simulink model "mecha_discrete_testing"  (R2016b)
settings: Solver=ode1  StartTime=0.0  StopTime=50  FixedStep=0.01  RelTol=1e-3
undefined symbols (not defined in the file or in its folder): DiscIntNeverNeededParam
libraries: dspinverses x1
settings Model: Creator=Utente  LastModifiedBy=Utente

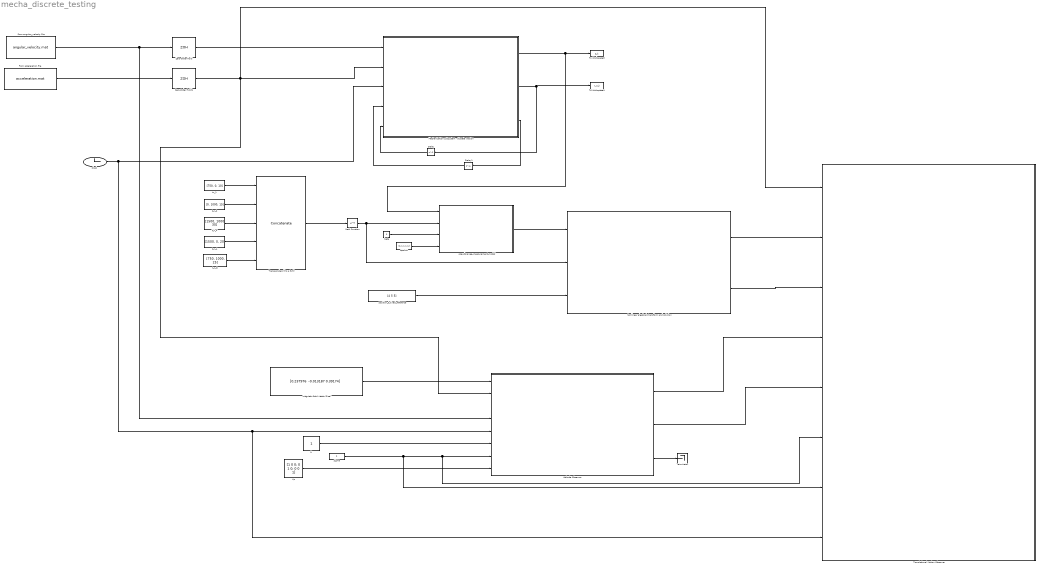
== system mecha_discrete_testing ==
  Attitude Observer : Subsystem
  Clock : Clock
      settings: Decimation=50
  Delay : Delay  DelayLength=1
  Delay1 : Delay  DelayLength=1
  From acceleration file : FromFile  FileName=acceleration.mat  SampleTime=0
  From angular_velocity file : FromFile  FileName=angular_velocity.mat  SampleTime=0
  Kp : Constant  Value=[1 0 0; 0 1 0; 0 0 1]
  Math Function : Math  Operator=transpose  SaturateOnIntegerOverflow=on
  Mechanisation subsystem - discrete version : Subsystem
  Nonlinear algebraic transform and solution : Subsystem
  Terminator : Terminator
  To Workspace3 : ToWorkspace  VariableName=p_k  SaveFormat=Timeseries  SampleTime=-1
  To Workspace4 : ToWorkspace  VariableName=v_n_k  SaveFormat=Timeseries  SampleTime=-1
  Translational Motion Observer : Subsystem
  Transponders (it's a 3x5) : Concatenate  NumInputs=5  Mode=Multidimensional array  ConcatenateDimension=2
  Zero-Order Hold : ZeroOrderHold  SampleTime=0.01
  Zero-Order Hold1 : ZeroOrderHold  SampleTime=0.01
  beta : Constant
  epsilon : Constant  Value=[1 1 1 1 1]
  ki : Constant
  magnetic field vector (Pisa) : Constant  Value="[0.237976  -0.013187 0.39174]"
  position_0_fixed_reference : Constant  Value=[4 5 5]
  pseudorange_measurement_model : MATLAB Function  TreatAsAtomicUnit=on
  sigma : Constant
  t_n_2 : Constant  Value=[0, 1000, 15]
  t_n_3 : Constant  Value=[1500, 1000, 30]
  t_n_4 : Constant  Value=[1500, 0, 20]
  t_n_5 : Constant  Value=[750, 1000, 25]
  tn_1 : Constant  Value=[750, 0, 10]
  wires:
  From acceleration file/1 -> Zero-Order Hold1/1
  From angular_velocity file/1 -> Attitude Observer/4(w_ib), Zero-Order Hold/1
  Zero-Order Hold/1 -> Mechanisation subsystem - discrete version/1(w_ib)
  Mechanisation subsystem - discrete version/1(p_n_k) -> pseudorange_measurement_model/1(p_n), To Workspace3/1
  Mechanisation subsystem - discrete version/3(R_nb_k_1) -> Delay1/1
  Mechanisation subsystem - discrete version/2(v_n_k_1) -> Delay/1, To Workspace4/1
  Delay/1 -> Mechanisation subsystem - discrete version/5(v_n_k)
  Delay1/1 -> Mechanisation subsystem - discrete version/4(R_nb_k)
  beta/1 -> pseudorange_measurement_model/3(beta)
  epsilon/1 -> pseudorange_measurement_model/4(epsilon)
  t_n_5/1 -> Transponders (it's a 3x5)/5
  t_n_4/1 -> Transponders (it's a 3x5)/4
  t_n_3/1 -> Transponders (it's a 3x5)/3
  t_n_2/1 -> Transponders (it's a 3x5)/2
  tn_1/1 -> Transponders (it's a 3x5)/1
  pseudorange_measurement_model/1(y) -> Nonlinear algebraic transform and solution/1(y)
  Math Function/1 -> Nonlinear algebraic transform and solution/2(p), pseudorange_measurement_model/2(p_n_i)
  Transponders (it's a 3x5)/1 -> Math Function/1
  position_0_fixed_reference/1 -> Nonlinear algebraic transform and solution/3(p0)
  Nonlinear algebraic transform and solution/2(C_dx) -> Translational Motion Observer/3(C_dx)
  Kp/1 -> Attitude Observer/8(Kp)
  sigma/1 -> Translational Motion Observer/7(Kp), Translational Motion Observer/6(sigma), Attitude Observer/7(sigma)
  ki/1 -> Attitude Observer/6(Ki)
  magnetic field vector (Pisa)/1 -> Attitude Observer/1(m_b_mag)
  Clock/1 -> Translational Motion Observer/8(t), Attitude Observer/5(t), Mechanisation subsystem - discrete version/3(t)
  Nonlinear algebraic transform and solution/1(delta) -> Translational Motion Observer/2(delta)
  Zero-Order Hold1/1 -> Translational Motion Observer/1(f_b_imu), Attitude Observer/2(f_b), Mechanisation subsystem - discrete version/2(f_b)
  Attitude Observer/1(J) -> Translational Motion Observer/4(J)
  Attitude Observer/2(R_nb_stim) -> Translational Motion Observer/5(R_nb_stim)
  Attitude Observer/3(b_stim) -> Terminator/1

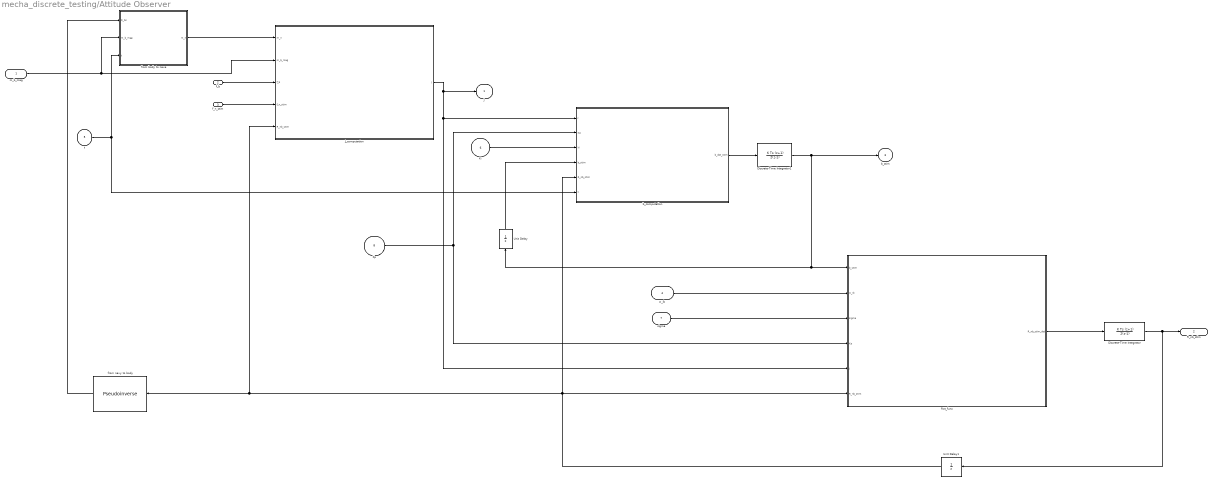
== system mecha_discrete_testing/Attitude Observer ==
  m_b_mag : Inport
  f_b : Inport  Port=2
  f_n_stim : Inport  Port=3
  w_ib : Inport  Port=4
  t : Inport  Port=5
  Ki : Inport  Port=6
  sigma : Inport  Port=7
  Kp : Inport  Port=8
  Discrete-Time Integrator : DiscreteIntegrator  IntegratorMethod=Integration: Trapezoidal  InitialConditionSetting=State (most efficient)  SampleTime=-1  ICPrevOutput=DiscIntNeverNeededParam  ICPrevScaledInput=DiscIntNeverNeededParam
  Discrete-Time Integrator1 : DiscreteIntegrator  IntegratorMethod=Integration: Trapezoidal  InitialConditionSetting=State (most efficient)  SampleTime=-1  ICPrevOutput=DiscIntNeverNeededParam  ICPrevScaledInput=DiscIntNeverNeededParam
  J_computation : Subsystem
  Rot_func : MATLAB Function  TreatAsAtomicUnit=on
  Unit Delay : UnitDelay  SampleTime=-1
  Unit Delay1 : UnitDelay  SampleTime=-1
  b_computation : MATLAB Function  TreatAsAtomicUnit=on
  from body to nave : MATLAB Function  TreatAsAtomicUnit=on
  from navy to body : dspinverses/Pseudoinverse  wanterr=off  SimulateUsing=Interpreted execution
  J : Outport
  R_nb_stim : Outport  Port=2
  b_stim : Outport  Port=3
  wires:
  m_b_mag/1 -> J_computation/2(m_b_mag), from body to nave/2(m_b_mag)
  Rot_func/1(R_nb_stim_dot) -> Discrete-Time Integrator/1
  b_computation/1(b_dot_stim) -> Discrete-Time Integrator1/1
  Discrete-Time Integrator1/1 -> b_stim/1, Unit Delay/1, Rot_func/1(b_stim)
  from body to nave/1(m_n) -> J_computation/1(m_n)
  f_b/1 -> J_computation/3(f_b)
  f_n_stim/1 -> J_computation/4(f_n_stim)
  J_computation/1(J) -> Rot_func/5(J), b_computation/1(J), J/1
  Kp/1 -> b_computation/2(Kp), Rot_func/4(Kp)
  Ki/1 -> b_computation/3(ki)
  sigma/1 -> Rot_func/3(sigma)
  w_ib/1 -> Rot_func/2(w_ib)
  t/1 -> b_computation/6(t), from body to nave/3(t)
  Discrete-Time Integrator/1 -> R_nb_stim/1, Unit Delay1/1
  Unit Delay/1 -> b_computation/4(b_stim)
  Unit Delay1/1 -> b_computation/5(R_nb_stim), Rot_func/6(R_nb_stim), J_computation/5(R_nb_stim), from navy to body/1
  from navy to body/1 -> from body to nave/1(R_bn)

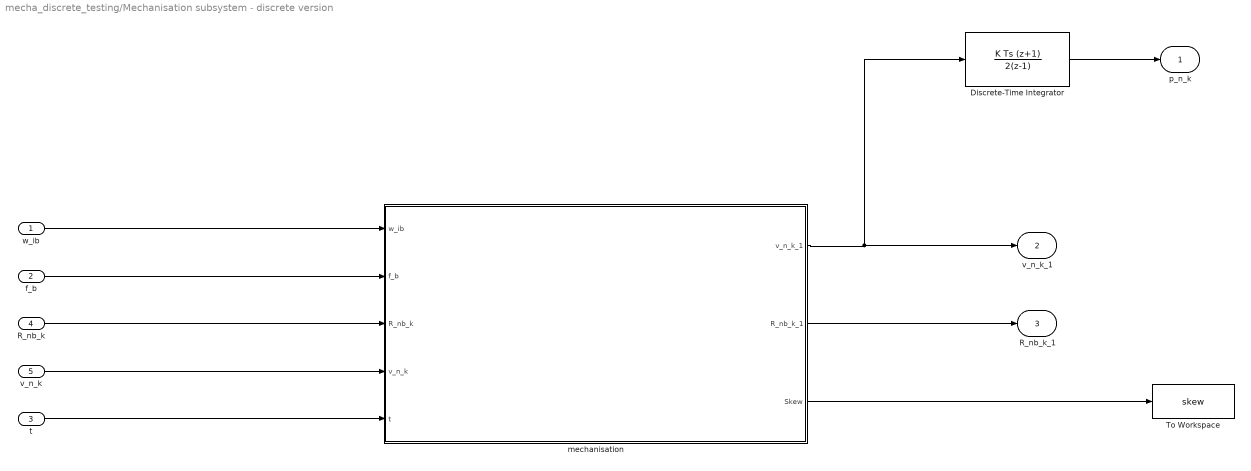
== system mecha_discrete_testing/Mechanisation subsystem - discrete version ==
  w_ib : Inport
  f_b : Inport  Port=2
  t : Inport  Port=3
  R_nb_k : Inport  Port=4
  v_n_k : Inport  Port=5
  Discrete-Time Integrator : DiscreteIntegrator  IntegratorMethod=Integration: Trapezoidal  InitialConditionSetting=State (most efficient)  SampleTime=-1  ICPrevOutput=DiscIntNeverNeededParam  ICPrevScaledInput=DiscIntNeverNeededParam
  To Workspace : ToWorkspace  VariableName=skew  SaveFormat=Timeseries  SampleTime=-1
  mechanisation : MATLAB Function  TreatAsAtomicUnit=on
  p_n_k : Outport
  v_n_k_1 : Outport  Port=2
  R_nb_k_1 : Outport  Port=3
  wires:
  w_ib/1 -> mechanisation/1(w_ib)
  t/1 -> mechanisation/5(t)
  f_b/1 -> mechanisation/2(f_b)
  Discrete-Time Integrator/1 -> p_n_k/1
  mechanisation/3(Skew) -> To Workspace/1
  mechanisation/1(v_n_k_1) -> v_n_k_1/1, Discrete-Time Integrator/1
  mechanisation/2(R_nb_k_1) -> R_nb_k_1/1
  R_nb_k/1 -> mechanisation/3(R_nb_k)
  v_n_k/1 -> mechanisation/4(v_n_k)

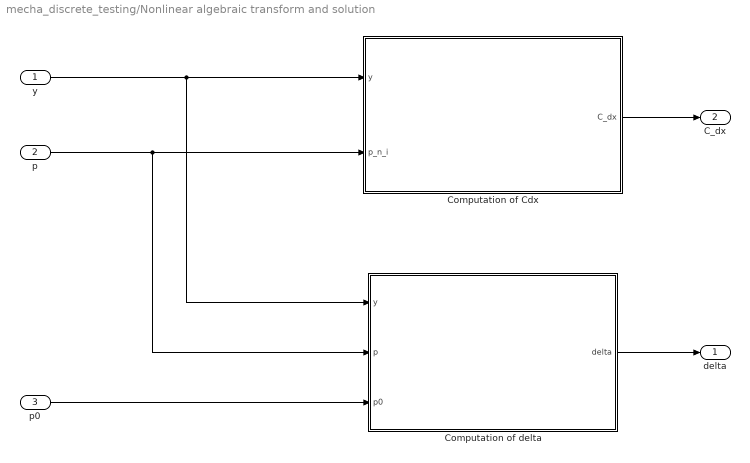
== system mecha_discrete_testing/Nonlinear algebraic transform and solution ==
  y : Inport
  p : Inport  Port=2
  p0 : Inport  Port=3
  Computation of Cdx : MATLAB Function  TreatAsAtomicUnit=on
  Computation of delta : MATLAB Function  TreatAsAtomicUnit=on
  delta : Outport
  C_dx : Outport  Port=2
  wires:
  y/1 -> Computation of delta/1(y), Computation of Cdx/1(y)
  p/1 -> Computation of delta/2(p), Computation of Cdx/2(p_n_i)
  p0/1 -> Computation of delta/3(p0)
  Computation of delta/1(delta) -> delta/1
  Computation of Cdx/1(C_dx) -> C_dx/1

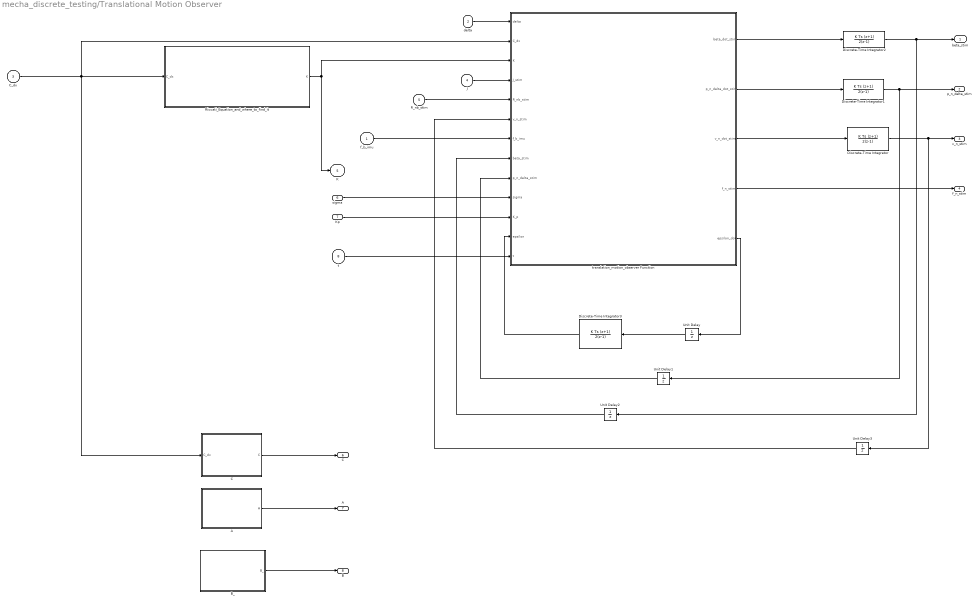
== system mecha_discrete_testing/Translational Motion Observer ==
  f_b_imu : Inport
  delta : Inport  Port=2
  C_dx : Inport  Port=3
  J : Inport  Port=4
  R_nb_stim : Inport  Port=5
  sigma : Inport  Port=6
  Kp : Inport  Port=7
  t : Inport  Port=8
  A : MATLAB Function  TreatAsAtomicUnit=on
  B_ : MATLAB Function  TreatAsAtomicUnit=on
  C : MATLAB Function  TreatAsAtomicUnit=on
  Discrete-Time Integrator{,1..3} (4 alike) : DiscreteIntegrator  IntegratorMethod=Integration: Trapezoidal  InitialConditionSetting=State (most efficient)  SampleTime=-1  ICPrevOutput=DiscIntNeverNeededParam  ICPrevScaledInput=DiscIntNeverNeededParam
  Riccati_Equation_and_where_to_find_it : Subsystem
  Unit Delay{,1..3} (4 alike) : UnitDelay  SampleTime=-1
  translation_motion_observer Function : MATLAB Function  TreatAsAtomicUnit=on
  beta_stim : Outport
  p_n_delta_stim : Outport  Port=2
  v_n_stim : Outport  Port=3
  f_n_stim : Outport  Port=4
  K : Outport  Port=5
  "C " : Outport  Port=6
  " A" : Outport  Port=7
  B : Outport  Port=8
  wires:
  translation_motion_observer Function/4(f_n_stim) -> f_n_stim/1
  translation_motion_observer Function/3(v_n_dot_stim) -> Discrete-Time Integrator/1
  Discrete-Time Integrator/1 -> Unit Delay3/1, v_n_stim/1
  translation_motion_observer Function/2(p_n_delta_dot_stim) -> Discrete-Time Integrator1/1
  Discrete-Time Integrator1/1 -> Unit Delay1/1, p_n_delta_stim/1
  Discrete-Time Integrator2/1 -> Unit Delay2/1, beta_stim/1
  translation_motion_observer Function/1(beta_dot_stim) -> Discrete-Time Integrator2/1
  translation_motion_observer Function/5(epsilon_dot) -> Unit Delay/1
  C_dx/1 -> C/1(C_dx), Riccati_Equation_and_where_to_find_it/1(C_dx), translation_motion_observer Function/2(C_dx)
  J/1 -> translation_motion_observer Function/4(J_stim)
  R_nb_stim/1 -> translation_motion_observer Function/5(R_nb_stim)
  delta/1 -> translation_motion_observer Function/1(delta)
  f_b_imu/1 -> translation_motion_observer Function/7(f_b_imu)
  sigma/1 -> translation_motion_observer Function/10(sigma)
  Kp/1 -> translation_motion_observer Function/11(K_p)
  A/1(A) -> " A"/1
  C/1(C) -> "C "/1
  Riccati_Equation_and_where_to_find_it/1(K) -> K/1, translation_motion_observer Function/3(K)
  B_/1(B_) -> B/1
  t/1 -> translation_motion_observer Function/13(t)
  Discrete-Time Integrator3/1 -> translation_motion_observer Function/12(epsilon)
  Unit Delay1/1 -> translation_motion_observer Function/9(p_n_delta_stim)
  Unit Delay2/1 -> translation_motion_observer Function/8(beta_stim)
  Unit Delay3/1 -> translation_motion_observer Function/6(v_n_stim)
  Unit Delay/1 -> Discrete-Time Integrator3/1

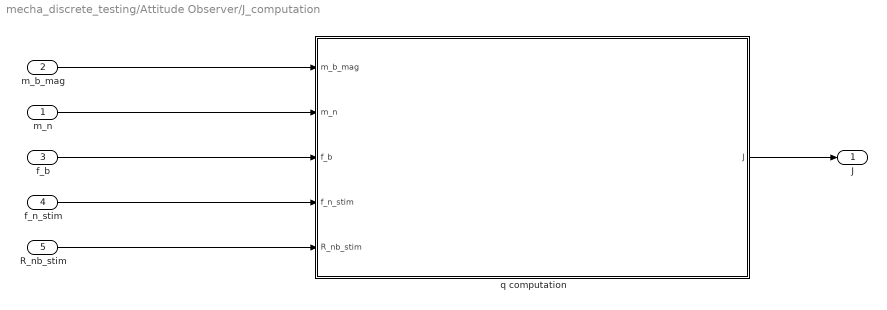
== system mecha_discrete_testing/Attitude Observer/J_computation ==
  m_n : Inport
  m_b_mag : Inport  Port=2
  f_b : Inport  Port=3
  f_n_stim : Inport  Port=4
  R_nb_stim : Inport  Port=5
  q computation : MATLAB Function  TreatAsAtomicUnit=on
  J : Outport
  wires:
  m_n/1 -> q computation/2(m_n)
  f_n_stim/1 -> q computation/4(f_n_stim)
  f_b/1 -> q computation/3(f_b)
  q computation/1(J) -> J/1
  R_nb_stim/1 -> q computation/5(R_nb_stim)
  m_b_mag/1 -> q computation/1(m_b_mag)

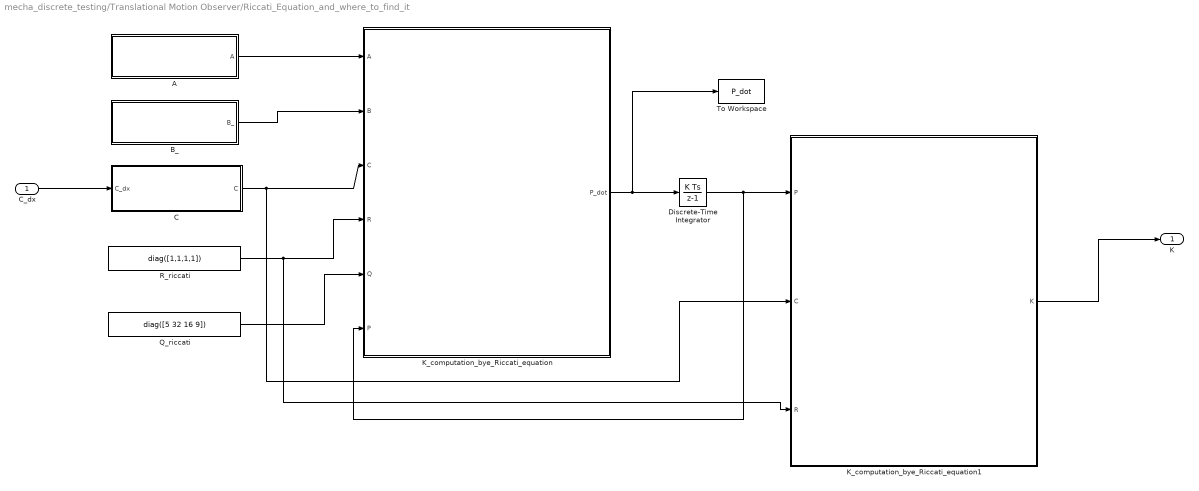
== system mecha_discrete_testing/Translational Motion Observer/Riccati_Equation_and_where_to_find_it ==
  C_dx : Inport
  A : MATLAB Function  TreatAsAtomicUnit=on
  B_ : MATLAB Function  TreatAsAtomicUnit=on
  C : MATLAB Function  TreatAsAtomicUnit=on
  Discrete-Time Integrator : DiscreteIntegrator  InitialConditionSetting=State (most efficient)  SampleTime=-1  ICPrevOutput=DiscIntNeverNeededParam  ICPrevScaledInput=DiscIntNeverNeededParam
  K_computation_bye_Riccati_equation : MATLAB Function  TreatAsAtomicUnit=on
  K_computation_bye_Riccati_equation1 : MATLAB Function  TreatAsAtomicUnit=on
  Q_riccati : Constant  Value=diag([5 32 16 9])
  R_riccati : Constant  Value=diag([1,1,1,1])
  To Workspace : ToWorkspace  VariableName=P_dot  SampleTime=-1
  K : Outport
  wires:
  C_dx/1 -> C/1(C_dx)
  R_riccati/1 -> K_computation_bye_Riccati_equation1/3(R), K_computation_bye_Riccati_equation/4(R)
  A/1(A) -> K_computation_bye_Riccati_equation/1(A)
  Q_riccati/1 -> K_computation_bye_Riccati_equation/5(Q)
  C/1(C) -> K_computation_bye_Riccati_equation1/2(C), K_computation_bye_Riccati_equation/3(C)
  B_/1(B_) -> K_computation_bye_Riccati_equation/2(B)
  K_computation_bye_Riccati_equation1/1(K) -> K/1
  K_computation_bye_Riccati_equation/1(P_dot) -> Discrete-Time Integrator/1, To Workspace/1
  Discrete-Time Integrator/1 -> K_computation_bye_Riccati_equation/6(P), K_computation_bye_Riccati_equation1/1(P)

== matlab function mecha_discrete_testing/Mechanisation subsystem - discrete version/mechanisation ==
  data: w_ib input; f_b input; v_n_k_1 output; R_nb_k_1 output; R_nb_k input size=[3,3]; v_n_k input size=[3,1]; t input; Skew output size=[3,3]
function [v_n_k_1, R_nb_k_1, Skew] = mechanisation(w_ib, f_b, R_nb_k, v_n_k, t)


Ts = 1/100; % sampling time
g_n = [0 0 9.81]';
 R_nb_z = zeros(3);

% ###############################

% init

if t == 0
    %v_n_k_1= ones(3,1);
    v_n_k = zeros(3,1);
   
    %R_nb_k_1 = eye(3);
    R_nb_k = eye(3);
    
   
end


% ###############################
% computing Skew matrix

% Skew = zeros(3,3);
% Skew(1,2) = -w_ib(3);
% Skew(2,1) = w_ib(3);
% Skew(1,3) = w_ib(2);
% Skew(3,1) = -w_ib(2);
% Skew(2,3) = -w_ib(1);
% Skew(3,2) = w_ib(1);

Skew = skew(w_ib);

% ###############################

% mechanisation

v_n_k_1 = Ts * ( R_nb_k * f_b + g_n) + v_n_k; 

if t ~=0
    R_nb_k_1 = Ts * R_nb_k * Skew + R_nb_k;
else
    R_nb_k_1 = Ts * R_nb_k * Skew + R_nb_z;
end

% ###############################

% updating

%v_n_k = v_n_k_1;

%R_nb_k = R_nb_k_1;
end

== matlab function mecha_discrete_testing/Attitude Observer/J_computation/q computation ==
  data: m_b_mag input; m_n input; f_b input; f_n_stim input size=3; J output; R_nb_stim input size=[3,3]
function J  = qEfunc(m_b_mag, m_n, f_b, f_n_stim, R_nb_stim)

g_n = [0 0 9.81]';

q1_b = m_b_mag/norm(m_b_mag,2);
q2_b = f_b/norm(g_n,2);

q1_n = m_n/norm(m_n,2);
q2_n = f_n_stim/norm(g_n,2);


E_b = [q1_b, skew(q1_b)*q2_b, (skew(q1_b)*skew(q1_b))*q2_b];
E_n = [q1_n, skew(q1_n)*q2_n, (skew(q1_n)*skew(q1_n))*q2_n];

J = (E_n - R_nb_stim * E_b) * (E_b');

end

== matlab function mecha_discrete_testing/Translational Motion Observer/Riccati_Equation_and_where_to_find_it/B_ ==
  data: B_ output
function B_ = B()

 B_ = zeros(10,3);

 B_(8:10,1:3) = eye(3);
end

== matlab function mecha_discrete_testing/Attitude Observer/b_computation ==
  data: J input; b_dot_stim output size=3; Kp input; ki input; b_stim input; R_nb_stim input; t input
function b_dot_stim = b_dot_stim_func(J, Kp, ki, b_stim, R_nb_stim, t)

%b_dot_stim = zeros(3 ,1);

if t == 0
    b_stim = zeros(3, 1);
end

SAT = sat(R_nb_stim)';
PA = pa( SAT * Kp * J);
VEX = vexfunc(PA);
b_dot_stim = Proj(b_stim , -ki * VEX);

end

== matlab function mecha_discrete_testing/Translational Motion Observer/translation_motion_observer Function ==
  data: delta input; C_dx input; K input; beta_dot_stim output; J_stim input; R_nb_stim input; p_n_delta_dot_stim output; v_n_dot_stim output; f_n_stim output size=[3,1]; v_n_stim input size=3; f_b_imu input size=3; beta_stim input; p_n_delta_stim input size=3; sigma input; K_p input; epsilon_dot output; epsilon input size=3; t input
function [beta_dot_stim,p_n_delta_dot_stim,v_n_dot_stim,f_n_stim,epsilon_dot] =  TMO_func(delta,C_dx,K,J_stim,R_nb_stim, v_n_stim,f_b_imu, beta_stim, p_n_delta_stim,sigma,K_p,epsilon,t)

 K_pp = K(1:3,:); 
 K_beta_p = K(4,:);
 K_v_p = K(5:7,:);
 K_eps_p = K(8:10,:);
 %obtained by Riccati equation..


% remember to insert a clock to define dimensions of all variables
g_n = [0 0 9.81]';

if(t == 0) 
   
    delta_stim = zeros(3, 1);
    delta_diff = zeros(3, 1);
    v_n_stim = zeros(3, 1);
    beta_stim = 0;
    epsilon = zeros(3,1);
    p_n_delta_stim = zeros(3, 1);
        
end



x_stim = [p_n_delta_stim; beta_stim];
%delta_stim = 2*C_dx*x_stim;
%delta_diff = (delta - delta_stim);



p_n_delta_dot_stim = v_n_stim + K_pp * (delta - 2*C_dx*x_stim);       % eq 14


beta_dot_stim = K_beta_p * (delta - 2*C_dx*x_stim);                       % eq 15


%theoretically we can't know epsilon
f_n_stim = R_nb_stim*f_b_imu + epsilon ;         % eq 18


v_n_dot_stim  = f_n_stim + g_n + K_v_p*(delta - 2*C_dx*x_stim);         % eq 16


epsilon_dot   = -sigma*K_p*J_stim*f_b_imu + K_eps_p*(delta - 2*C_dx*x_stim); % eq 17
end

== matlab function mecha_discrete_testing/Nonlinear algebraic transform and solution/Computation of Cdx ==
  data: y input; p_n_i input; C_dx output size=[4,4]
function C_dx  = C_dx_func(y,p_n_i)

    % y vector 
    % p matrix has row vectors
    %            (x,y,z) cols 
    %            m-rows are transponders number
    % all variables are in navigation frame oh yeah! baby ;)
    
    % vorsicht
    % both y and p_n_i (i=1,...,m) are column vectors   
    
    [row_,col_] = size(y);
    [row,col] = size(p_n_i);
    
    % taking the m-th vecotr both for y and p_n_i
    % I've to choose one measurement as referement at each sample time, so
    % a reference transponder
    % since y is a row vector
    
    y_m = y(row_);
    p_m = p_n_i(row,:);
    
    % row_ and row may be eqaul

    m = row; % m is the number of measurement at one step, so eqaul to the number of transponders
    
    % let's build the vector that will fill the matrix C_dx
    
    y_ = zeros(m-1,1);
    p_ = zeros(m-1,3); %row vector, 3 stands for x,y,z
    
    
    for i = 1 : 1 : m-1
    
        y_(i) = y(i) - y_m;
        
        p_(i,:) = p_m - p_n_i(i,:);    
        
    end
    
    % building matrix C_dx
    
    C_dx = [p_, y_]; % (m-1)x4

end

== matlab function mecha_discrete_testing/Nonlinear algebraic transform and solution/Computation of delta ==
  data: y input; delta output size=4; p input; p0 input
function delta  = delta_func(y,p,p0)

    % p is 5x3
    % note that here p is the same of p_n_i of the other function in this
    % subsystem

    % y vector 
    % p matrix has row vectors
    %            (x,y,z) cols 
    %            m-rows are the numbers of the transponders
    % all variables are in navigation frame oh yeah! baby ;)
    % z is a col vector of scalars
    
    % we must choose p0 (a block)
    % p0 is a column vector (3x1)
    
    [row,col] = size(p); %5x3 here since we have 5 transponders
    %[row_,col_] = size(y);
    
    % building line-of-sight vector
    p_los = zeros(row,col);
    z = zeros(row,1);
    %defining los vector
    
    % computing line-of-sigth vectors
    for i=1:1:row
       p_los(i,:) = p(i,:) - p0';
    end
    
    % p_los is 5x3 ...
    p_los = p_los';
    % now 3x5

    for i = 1:1:row
        z(i,1)= (y(i)^2 - norm(p_los(:,i))^2);
    end

    z = z'; % now a row vector

    delta = zeros(row-1,1);
    
    z_m = z(end);

    for i = 1:1:row-1
        delta(i,1) =  (z(i) - z_m);
    end

    delta; % a column vector

end

== matlab function mecha_discrete_testing/Translational Motion Observer/Riccati_Equation_and_where_to_find_it/K_computation_bye_Riccati_equation ==
  data: A input; B input; P_dot output; C input; R input; Q input; P input size=[10, 10]
function P_dot = P_dot_func(A,B,C,R,Q,P)

%K = zeros(10,3);

%coder.extrinsic('care');

Q_ = C'*Q*C;

%[P,L,G] = care(A,C',Q_,R);

R_inv = pinv(R); 

P_dot = P*A + A' * P - P*C'*R_inv*C*P + Q_;

%K = P*C'*R_inv;

end

== matlab function mecha_discrete_testing/Translational Motion Observer/Riccati_Equation_and_where_to_find_it/A ==
  data: A output
function A = A()

 A = zeros(10);

 A(1:3,5:7) = eye(3);
 A(5:7,8:10) = eye(3);
 
end

== matlab function mecha_discrete_testing/Translational Motion Observer/Riccati_Equation_and_where_to_find_it/C ==
  data: C output; C_dx input
function C = C(C_dx)

   row = size(C_dx,1); 

   C1 = zeros(row,6);

 C = [2*C_dx C1];

== matlab function mecha_discrete_testing/Attitude Observer/Rot_func ==
  data: b_stim input; R_nb_stim_dot output; w_ib input; sigma input; Kp input; J input; R_nb_stim input
function R_nb_stim_dot = rot_func(b_stim,w_ib,sigma,Kp,J,R_nb_stim) 

Skew = skew(w_ib - b_stim);

R_nb_stim_dot = R_nb_stim * Skew + sigma * Kp * J;

== matlab function mecha_discrete_testing/Translational Motion Observer/A ==
  data: A output
function A = A()

 A = zeros(10);

 A(1:3,5:7) = eye(3);
 A(5:7,8:10) = eye(3);
 
end

== matlab function mecha_discrete_testing/Translational Motion Observer/C ==
  data: C output; C_dx input
function C = Cfunc(C_dx)

   row = size(C_dx,1); 

   C1 = zeros(row,6);

 C = [2*C_dx C1];
 
 
end

== matlab function mecha_discrete_testing/Translational Motion Observer/B_ ==
  data: B_ output
function B_ = B()

 B_ = zeros(10,3);

 B_(8:10,1:3) = eye(3);
end

== matlab function mecha_discrete_testing/pseudorange_measurement_model ==
  data: p_n input; y output size=5; p_n_i input; beta input; epsilon input
function y = pseudorange_mea_model(p_n, p_n_i, beta, epsilon)

    % vorsicht
    % p_n_i are the transponder position in world frame
    % p_n_i here is a   5x3
    
  % we want to build y as a column vector so  
  y = zeros(size(p_n_i,1),1);

  for i = 1:1:size(p_n_i,1)

      rho = norm(p_n - p_n_i(i,:)');  % eq. 7 % norm 2
      
      y(i,1) = rho + beta + epsilon(i); % eq. 8 

  end
      
end

== matlab function mecha_discrete_testing/Translational Motion Observer/Riccati_Equation_and_where_to_find_it/K_computation_bye_Riccati_equation1 ==
  data: P input; K output; C input; R input
function K = K_func(P, C, R)

K = zeros(10,size(C,1));

R_inv = pinv(R);

K = P*C'*R_inv;

end

== matlab function mecha_discrete_testing/Attitude Observer/from body to nave ==
  data: R_bn input; m_n output; m_b_mag input; t input
function m_n = b2n(R_bn, m_b_mag,t)

if t==0
    R_bn = eye(3);
end

m_n = R_bn * m_b_mag;
